simulink library "predictor_lib"  (R2016b)
settings: Solver=ode45  StartTime=0.0  StopTime=10.0  RelTol=1e-3  EnableMultiTasking=on
undefined symbols (not defined in the file): A_B_ISS_ISS, accel_bias, ase_of_num_aug, ase_total_num_states, ase_ts, gyro_bias, omega_B_ISS_B, P_EST_ISS_ISS, quat_ISS2B, tun_ase_max_accel, tun_ase_max_gyro, tun_ase_Q_imu, tun_ase_q_saturated_accel, tun_ase_q_saturated_gyro, V_B_ISS_ISS
libraries: math_utils x3
settings Model: Creator=jfusco1  LastModifiedBy=jfusco1
settings DataIOCC: LimitDataPoints=on  SaveFormat=Array
settings OptimizationCC: LifeSpan=inf
settings DebuggingCC: AllowSymbolicDim=off  SFUnexpectedBacktrackingDiag=warning  SFNoUnconditionalDefaultTransitionDiag=warning  SFExecutionAtInitializationDiag=none
settings HardwareCC: ProdBitPerPointer=32  ProdBitPerSizeT=32  ProdBitPerPtrDiffT=32  ProdLargestAtomicFloat=None  ProdIntDivRoundTo=Undefined  ProdEndianess=Unspecified  ProdWordSize=32  ProdHWDeviceType=32-bit Generic
settings ModelReferenceCC: PropagateSignalLabelsOutOfModel=off
settings GRTTargetCC: TargetLangStandard=C89/C90 (ANSI)  GeneratePreprocessorConditionals=Disable all
settings ConfigComp: CovMetricSettings=dw  CovHtmlReporting=on  CovSaveCumulativeToWorkspaceVar=on  CovSaveSingleToWorkspaceVar=on  CovExternalEMLEnable=off

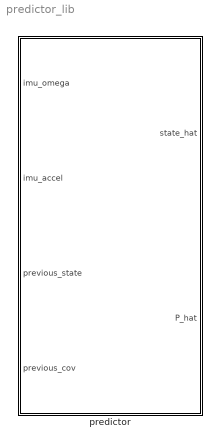
== system predictor_lib ==
  predictor : Subsystem

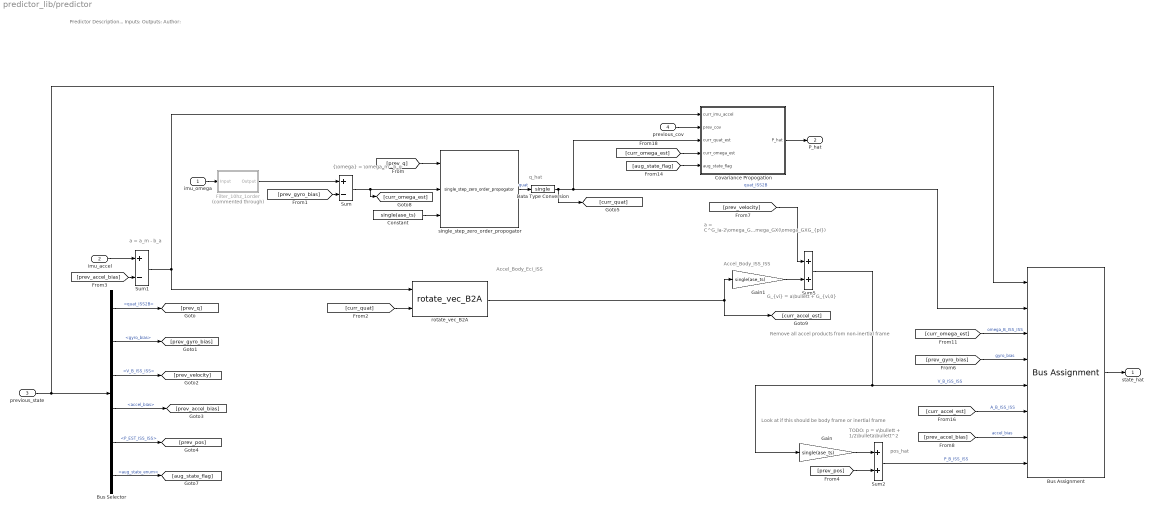
== system predictor_lib/predictor ==
  note: {\omega} = \omega_m - b_g
  note: Predictor
      | Description...
      |
      | Inputs:
      |
      | Outputs:
      |
      | Author:
  note: a = a_m - b_a
  note: q_hat
  note: TODO: p = v\bullett + 1/2\bulleta\bullett^2
  note: pos_hat
  note: a = C^G_Ia-2\omega_GXG_{vi}-\omega_GX(\omega_GXG_{pi})
  note: Accel_Body_Eci_ISS
  note: G_{vi} = a\bullett + G_{vi,0}
  note: Look at if this should be body frame or inertial frame
  note: Remove all accel products
      | from non-inertial frame
  note: Accel_Body_ISS_ISS
  imu_omega : Inport
  imu_accel : Inport  Port=2
  previous_state : Inport  Port=3
  previous_cov : Inport  Port=4
  Bus Assignment : BusAssignment  AssignedSignals=quat_ISS2B,omega_B_ISS_B,gyro_bias,V_B_ISS_ISS,A_B_ISS_ISS,accel_bias,P_EST_ISS_ISS
  Bus Selector : BusSelector  OutputSignals=quat_ISS2B,gyro_bias,V_B_ISS_ISS,accel_bias,P_EST_ISS_ISS,aug_state_enum
  Constant : Constant  Value=single(ase_ts)
  Covariance Propogation : Subsystem
  Data Type Conversion : DataTypeConversion  OutDataTypeStr=single
  Filter_10hz_1order : Subsystem  Tag=FilterWizardSubSystem  Commented=through
      settings: ErrorFcn=dspFilterRealizedInBasicElemsAlgLoopErrFcnCallback
  Gain : Gain  Gain=single(ase_ts)  OutDataTypeStr=single
  Gain1 : Gain  Gain=single(ase_ts)  OutDataTypeStr=single
  Sum : Sum  Inputs=+-
  Sum1 : Sum  Inputs=+-
  Sum2 : Sum
  Sum5 : Sum
  rotate_vec_B2A : math_utils/rotate_vec_B2A  SystemSampleTime=-1
  single_step_zero_order_propogator : math_utils/single_step_zero_order_propogator  SystemSampleTime=-1
  state_hat : Outport
  P_hat : Outport  Port=2
  wires:
  Bus Selector/4 -> [prev_accel_bias]  "<accel_bias>"
  Bus Selector/6 -> [aug_state_flag]  "<aug_state_enum>"
  Bus Assignment/1 -> state_hat/1
  imu_accel/1 -> Sum1/1
  Filter_10hz_1order/1(Output) -> Sum/1
  imu_omega/1 -> Filter_10hz_1order/1(Input)
  Sum/1 -> single_step_zero_order_propogator/2, [curr_omega_est]
  Constant/1 -> single_step_zero_order_propogator/3
  Gain/1 -> Sum2/1
  Sum1/1 -> rotate_vec_B2A/1, Covariance Propogation/1(curr_imu_accel)
  rotate_vec_B2A/1 -> Gain1/1, [curr_accel_est]
  Gain1/1 -> Sum5/2
  Bus Selector/1 -> [prev_q]  "<quat_ISS2B>"
  Bus Selector/2 -> [prev_gyro_bias]  "<gyro_bias>"
  Bus Selector/3 -> [prev_velocity]  "<V_B_ISS_ISS>"
  Bus Selector/5 -> [prev_pos]  "<P_EST_ISS_ISS>"
  [prev_q] -> single_step_zero_order_propogator/1
  [curr_quat] -> rotate_vec_B2A/2
  [prev_gyro_bias] -> Sum/2
  [prev_velocity] -> Sum5/1
  [prev_accel_bias] -> Sum1/2
  [prev_pos] -> Sum2/2
  single_step_zero_order_propogator/1 -> Data Type Conversion/1  "quat"
  [prev_accel_bias] -> Bus Assignment/7  "accel_bias"
  Sum2/1 -> Bus Assignment/8  "P_B_ISS_ISS"
  [prev_gyro_bias] -> Bus Assignment/4  "gyro_bias"
  Sum5/1 -> Bus Assignment/5, Gain/1  "V_B_ISS_ISS"
  Data Type Conversion/1 -> Covariance Propogation/3(curr_quat_est), Bus Assignment/2, [curr_quat]  "quat_ISS2B"
  previous_state/1 -> Bus Assignment/1, Bus Selector/1
  [curr_omega_est] -> Bus Assignment/3  "omega_B_ISS_ISS"
  [curr_accel_est] -> Bus Assignment/6  "A_B_ISS_ISS"
  previous_cov/1 -> Covariance Propogation/2(prev_cov)
  Covariance Propogation/1(P_hat) -> P_hat/1
  [curr_omega_est] -> Covariance Propogation/4(curr_omega_est)
  [aug_state_flag] -> Covariance Propogation/5(aug_state_flag)

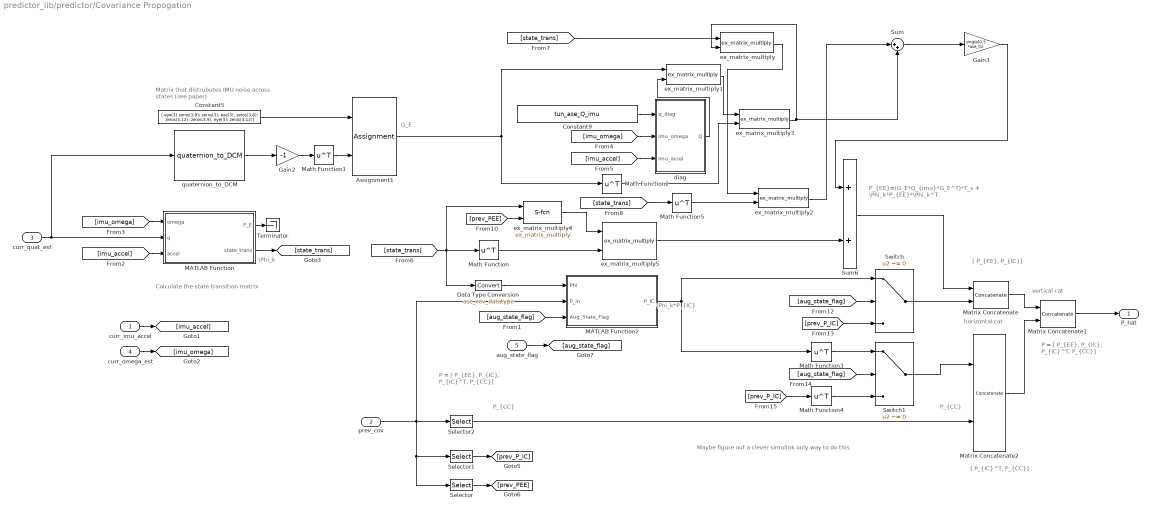
== system predictor_lib/predictor/Covariance Propogation ==
  note: P = [ P_{EE}, P_{IC};
      |
      |         P_{IC}^T, P_{CC}]
  note: \Phi_k
  note: G_E
  note: Matrix that distrubutes IMU noise across states (see paper)
  note: Calculate the state transition matrix
  note: P_{EE}=(G_E*Q_{imu}*G_E^T)*T_s + \Phi_k*P_{EE}*\Phi_k^T
  note: \Phi_k*P_{IC}
  note: P_{CC}
  note: P_{CC}
  note: [ P_{EE}, P_{IC}]
  note: [ P_{IC}^T, P_{CC}]
  note: P = [ P_{EE}, P_{IC};
      |
      |         P_{IC}^T, P_{CC}]
  note: horizontal cat
  note: vertical cat
  note: Maybe figure out a clever simulink only way to do this
  curr_imu_accel : Inport
  prev_cov : Inport  Port=2  OutDataTypeStr=ase_cov_datatype
  curr_quat_est : Inport  Port=3
  curr_omega_est : Inport  Port=4
  aug_state_flag : Inport  Port=5
  Assignment1 : Assignment  NumberOfDimensions=2  DiagnosticForDimensions=Warning  IndexOptions=Index vector (dialog),Index vector (dialog)  Indices=[7 8 9],[7 8 9]  OutputSizes=1,1
  Constant5 : Constant  Value=[-eye(3) zeros(3,9); zeros(3), eye(3), zeros(3,6); zeros(3,12); zeros(3,9), eye(3); zeros(3,12)]  OutDataTypeStr=ase_cov_datatype
  Constant9 : Constant  Value=tun_ase_Q_imu  OutDataTypeStr=ase_cov_datatype
  Data Type Conversion : DataTypeConversion  OutDataTypeStr=ase_cov_datatype
  Gain2 : Gain  Gain=-1  OutDataTypeStr=Inherit: Inherit via back propagation
  Gain3 : Gain  Gain=single(0.5 *ase_ts)
  MATLAB Function : MATLAB Function  TreatAsAtomicUnit=on
  MATLAB Function2 : MATLAB Function  TreatAsAtomicUnit=on
  Math Function{,1..5} (6 alike) : Math  Operator=transpose  SaturateOnIntegerOverflow=on
  Matrix Concatenate : Concatenate  Mode=Multidimensional array  ConcatenateDimension=2
  Matrix Concatenate1 : Concatenate  Mode=Multidimensional array
  Matrix Concatenate2 : Concatenate  Mode=Multidimensional array  ConcatenateDimension=2
  Selector : Selector  NumberOfDimensions=2  InputPortWidth=21  IndexOptions=Index vector (dialog),Index vector (dialog)  Indices=[1:15],[1:15]  OutputSizes=1,1
  Selector1 : Selector  NumberOfDimensions=2  InputPortWidth=21  IndexOptions=Index vector (dialog),Index vector (dialog)  Indices=[1:15],[16:ase_total_num_states]  OutputSizes=1,1
  Selector2 : Selector  NumberOfDimensions=2  InputPortWidth=21  IndexOptions=Index vector (dialog),Index vector (dialog)  Indices=[16:ase_total_num_states],[16:ase_total_num_states]  OutputSizes=1,1
  Sum : Sum  Inputs=|++
  Sum6 : Sum
  Switch : Switch  Criteria=u2 ~= 0
  Switch1 : Switch  Criteria=u2 ~= 0
  Terminator : Terminator
  diag : MATLAB Function  TreatAsAtomicUnit=on
  ex_matrix_multiply : S-Function  FunctionName=ex_matrix_multiply  SFunctionDeploymentMode=off  EnableBusSupport=off  mask(Legacy Function){SFunctionSpec=void matrix_multiply(single u1[][], int32 size(u1, 1), int32 size(u1, 2), single u2[][], int32 size(u2, 1), int32 size(u2, 2), single y1[size(u1, 1)][size(u2, 2)]), ShowSpec=off}
      mask prompts: ShowSpec "Display function specification"
      mask help:
      | This block allows you to call the legacy functions specified by the following Legacy Code Tool definition:
      | def.SFunctionName = 'ex_matrix_multiply';
      | def.OutputFcnSpec = 'void matrix_multiply(single u1[][], int32 size(u1, 1), int32 size(u1, 2), single u2[][], int32 size(u2, 1), int32 size(u2, 2), single y1[size(u1, 1)][size(u2, 2)])';
      | def.HeaderFiles = {'matrix_multiply.h'};
      | def.SourceFiles = {'matrix_multiply.cpp'};
      | def.IncPaths = {'cxx_functions/include', '/usr/include/eigen3'};
      | def.SrcPaths = {'cxx_functions/src', '/usr/include/eigen3/Eigen/src'};
      | def.Options.language = 'C++';
      mask Help: <p>This block was generated automatically by the Legacy Code Tool. For detailed help on this tool, call<a href="matlab:legacy_code('help')"> legacy_code('help')</a>.</p>
      mask Callback ShowSpec:
      | if strcmp(get_param(gcbh, 'ShowSpec'), 'on')
      |   set_param(gcbh, 'MaskDisplay', sprintf('fprintf(''%s'');', get_param(gcbh, 'SFunctionSpec')));
      | else
      |   set_param(gcbh, 'MaskDisplay', sprintf('fprintf(''%s'');', get_param(gcbh, 'FunctionName')));
      | end
      mask Display: fprintf('ex_matrix_multiply');
  ex_matrix_multiply1 : S-Function  FunctionName=ex_matrix_multiply  SFunctionDeploymentMode=off  EnableBusSupport=off  mask(Legacy Function){SFunctionSpec=void matrix_multiply(single u1[][], int32 size(u1, 1), int32 size(u1, 2), single u2[][], int32 size(u2, 1), int32 size(u2, 2), single y1[size(u1, 1)][size(u2, 2)]), ShowSpec=off}
      mask prompts: ShowSpec "Display function specification"
      mask help:
      | This block allows you to call the legacy functions specified by the following Legacy Code Tool definition:
      | def.SFunctionName = 'ex_matrix_multiply';
      | def.OutputFcnSpec = 'void matrix_multiply(single u1[][], int32 size(u1, 1), int32 size(u1, 2), single u2[][], int32 size(u2, 1), int32 size(u2, 2), single y1[size(u1, 1)][size(u2, 2)])';
      | def.HeaderFiles = {'matrix_multiply.h'};
      | def.SourceFiles = {'matrix_multiply.cpp'};
      | def.IncPaths = {'cxx_functions/include', '/usr/include/eigen3'};
      | def.SrcPaths = {'cxx_functions/src', '/usr/include/eigen3/Eigen/src'};
      | def.Options.language = 'C++';
      mask Help: <p>This block was generated automatically by the Legacy Code Tool. For detailed help on this tool, call<a href="matlab:legacy_code('help')"> legacy_code('help')</a>.</p>
      mask Callback ShowSpec:
      | if strcmp(get_param(gcbh, 'ShowSpec'), 'on')
      |   set_param(gcbh, 'MaskDisplay', sprintf('fprintf(''%s'');', get_param(gcbh, 'SFunctionSpec')));
      | else
      |   set_param(gcbh, 'MaskDisplay', sprintf('fprintf(''%s'');', get_param(gcbh, 'FunctionName')));
      | end
      mask Display: fprintf('ex_matrix_multiply');
  ex_matrix_multiply2 : S-Function  FunctionName=ex_matrix_multiply  SFunctionDeploymentMode=off  EnableBusSupport=off  mask(Legacy Function){SFunctionSpec=void matrix_multiply(single u1[][], int32 size(u1, 1), int32 size(u1, 2), single u2[][], int32 size(u2, 1), int32 size(u2, 2), single y1[size(u1, 1)][size(u2, 2)]), ShowSpec=off}
      mask prompts: ShowSpec "Display function specification"
      mask help:
      | This block allows you to call the legacy functions specified by the following Legacy Code Tool definition:
      | def.SFunctionName = 'ex_matrix_multiply';
      | def.OutputFcnSpec = 'void matrix_multiply(single u1[][], int32 size(u1, 1), int32 size(u1, 2), single u2[][], int32 size(u2, 1), int32 size(u2, 2), single y1[size(u1, 1)][size(u2, 2)])';
      | def.HeaderFiles = {'matrix_multiply.h'};
      | def.SourceFiles = {'matrix_multiply.cpp'};
      | def.IncPaths = {'cxx_functions/include', '/usr/include/eigen3'};
      | def.SrcPaths = {'cxx_functions/src', '/usr/include/eigen3/Eigen/src'};
      | def.Options.language = 'C++';
      mask Help: <p>This block was generated automatically by the Legacy Code Tool. For detailed help on this tool, call<a href="matlab:legacy_code('help')"> legacy_code('help')</a>.</p>
      mask Callback ShowSpec:
      | if strcmp(get_param(gcbh, 'ShowSpec'), 'on')
      |   set_param(gcbh, 'MaskDisplay', sprintf('fprintf(''%s'');', get_param(gcbh, 'SFunctionSpec')));
      | else
      |   set_param(gcbh, 'MaskDisplay', sprintf('fprintf(''%s'');', get_param(gcbh, 'FunctionName')));
      | end
      mask Display: fprintf('ex_matrix_multiply');
  ex_matrix_multiply3 : S-Function  FunctionName=ex_matrix_multiply  SFunctionDeploymentMode=off  EnableBusSupport=off  mask(Legacy Function){SFunctionSpec=void matrix_multiply(single u1[][], int32 size(u1, 1), int32 size(u1, 2), single u2[][], int32 size(u2, 1), int32 size(u2, 2), single y1[size(u1, 1)][size(u2, 2)]), ShowSpec=off}
      mask prompts: ShowSpec "Display function specification"
      mask help:
      | This block allows you to call the legacy functions specified by the following Legacy Code Tool definition:
      | def.SFunctionName = 'ex_matrix_multiply';
      | def.OutputFcnSpec = 'void matrix_multiply(single u1[][], int32 size(u1, 1), int32 size(u1, 2), single u2[][], int32 size(u2, 1), int32 size(u2, 2), single y1[size(u1, 1)][size(u2, 2)])';
      | def.HeaderFiles = {'matrix_multiply.h'};
      | def.SourceFiles = {'matrix_multiply.cpp'};
      | def.IncPaths = {'cxx_functions/include', '/usr/include/eigen3'};
      | def.SrcPaths = {'cxx_functions/src', '/usr/include/eigen3/Eigen/src'};
      | def.Options.language = 'C++';
      mask Help: <p>This block was generated automatically by the Legacy Code Tool. For detailed help on this tool, call<a href="matlab:legacy_code('help')"> legacy_code('help')</a>.</p>
      mask Callback ShowSpec:
      | if strcmp(get_param(gcbh, 'ShowSpec'), 'on')
      |   set_param(gcbh, 'MaskDisplay', sprintf('fprintf(''%s'');', get_param(gcbh, 'SFunctionSpec')));
      | else
      |   set_param(gcbh, 'MaskDisplay', sprintf('fprintf(''%s'');', get_param(gcbh, 'FunctionName')));
      | end
      mask Display: fprintf('ex_matrix_multiply');
  ex_matrix_multiply4 : S-Function  FunctionName=ex_matrix_multiply  SFunctionDeploymentMode=off  EnableBusSupport=off  mask(Legacy Function){SFunctionSpec=void matrix_multiply(single u1[][], int32 size(u1, 1), int32 size(u1, 2), single u2[][], int32 size(u2, 1), int32 size(u2, 2), single y1[size(u1, 1)][size(u2, 2)]), ShowSpec=off}
      mask prompts: ShowSpec "Display function specification"
      mask help:
      | This block allows you to call the legacy functions specified by the following Legacy Code Tool definition:
      | def.SFunctionName = 'ex_matrix_multiply';
      | def.OutputFcnSpec = 'void matrix_multiply(single u1[][], int32 size(u1, 1), int32 size(u1, 2), single u2[][], int32 size(u2, 1), int32 size(u2, 2), single y1[size(u1, 1)][size(u2, 2)])';
      | def.HeaderFiles = {'matrix_multiply.h'};
      | def.SourceFiles = {'matrix_multiply.cpp'};
      | def.IncPaths = {'cxx_functions/include', '/usr/include/eigen3'};
      | def.SrcPaths = {'cxx_functions/src', '/usr/include/eigen3/Eigen/src'};
      | def.Options.language = 'C++';
      mask Help: <p>This block was generated automatically by the Legacy Code Tool. For detailed help on this tool, call<a href="matlab:legacy_code('help')"> legacy_code('help')</a>.</p>
      mask Callback ShowSpec:
      | if strcmp(get_param(gcbh, 'ShowSpec'), 'on')
      |   set_param(gcbh, 'MaskDisplay', sprintf('fprintf(''%s'');', get_param(gcbh, 'SFunctionSpec')));
      | else
      |   set_param(gcbh, 'MaskDisplay', sprintf('fprintf(''%s'');', get_param(gcbh, 'FunctionName')));
      | end
      mask Display: fprintf('ex_matrix_multiply');
  ex_matrix_multiply5 : S-Function  FunctionName=ex_matrix_multiply  SFunctionDeploymentMode=off  EnableBusSupport=off  mask(Legacy Function){SFunctionSpec=void matrix_multiply(single u1[][], int32 size(u1, 1), int32 size(u1, 2), single u2[][], int32 size(u2, 1), int32 size(u2, 2), single y1[size(u1, 1)][size(u2, 2)]), ShowSpec=off}
      mask prompts: ShowSpec "Display function specification"
      mask help:
      | This block allows you to call the legacy functions specified by the following Legacy Code Tool definition:
      | def.SFunctionName = 'ex_matrix_multiply';
      | def.OutputFcnSpec = 'void matrix_multiply(single u1[][], int32 size(u1, 1), int32 size(u1, 2), single u2[][], int32 size(u2, 1), int32 size(u2, 2), single y1[size(u1, 1)][size(u2, 2)])';
      | def.HeaderFiles = {'matrix_multiply.h'};
      | def.SourceFiles = {'matrix_multiply.cpp'};
      | def.IncPaths = {'cxx_functions/include', '/usr/include/eigen3'};
      | def.SrcPaths = {'cxx_functions/src', '/usr/include/eigen3/Eigen/src'};
      | def.Options.language = 'C++';
      mask Help: <p>This block was generated automatically by the Legacy Code Tool. For detailed help on this tool, call<a href="matlab:legacy_code('help')"> legacy_code('help')</a>.</p>
      mask Callback ShowSpec:
      | if strcmp(get_param(gcbh, 'ShowSpec'), 'on')
      |   set_param(gcbh, 'MaskDisplay', sprintf('fprintf(''%s'');', get_param(gcbh, 'SFunctionSpec')));
      | else
      |   set_param(gcbh, 'MaskDisplay', sprintf('fprintf(''%s'');', get_param(gcbh, 'FunctionName')));
      | end
      mask Display: fprintf('ex_matrix_multiply');
  quaternion_to_DCM : math_utils/quaternion_to_DCM  SystemSampleTime=-1
  P_hat : Outport  OutDataTypeStr=ase_cov_datatype
  wires:
  ex_matrix_multiply1/1 -> ex_matrix_multiply3/1
  ex_matrix_multiply4/1 -> ex_matrix_multiply5/1
  Math Function5/1 -> ex_matrix_multiply2/2
  [state_trans] -> Math Function5/1
  [state_trans] -> ex_matrix_multiply/1
  [state_trans] -> Math Function/1, Data Type Conversion/1, ex_matrix_multiply4/1
  MATLAB Function/2(state_trans) -> [state_trans]
  [imu_accel] -> diag/3(imu_accel)
  [imu_omega] -> diag/2(imu_omega)
  [imu_omega] -> MATLAB Function/1(omega)
  curr_omega_est/1 -> [imu_omega]
  [imu_accel] -> MATLAB Function/3(accel)
  curr_imu_accel/1 -> [imu_accel]
  diag/1(Q) -> ex_matrix_multiply1/2
  Data Type Conversion/1 -> MATLAB Function2/1(Phi)
  prev_cov/1 -> Selector/1, Selector1/1, Selector2/1, MATLAB Function2/2(P_in)
  [aug_state_flag] -> MATLAB Function2/3(Aug_State_Flag)
  [prev_P_IC] -> Switch/3
  Matrix Concatenate2/1 -> Matrix Concatenate1/2
  Selector/1 -> [prev_PEE]
  [aug_state_flag] -> Switch1/2
  Selector2/1 -> Matrix Concatenate2/2
  Selector1/1 -> [prev_P_IC]
  [aug_state_flag] -> Switch/2
  MATLAB Function2/1(P_IC) -> Switch/1, Math Function3/1
  ex_matrix_multiply3/1 -> Sum/2, ex_matrix_multiply/2
  Matrix Concatenate/1 -> Matrix Concatenate1/1
  Matrix Concatenate1/1 -> P_hat/1
  Switch/1 -> Matrix Concatenate/2
  Switch1/1 -> Matrix Concatenate2/1
  Math Function3/1 -> Switch1/1
  Constant5/1 -> Assignment1/1
  Sum6/1 -> Matrix Concatenate/1
  Assignment1/1 -> Math Function2/1, ex_matrix_multiply1/1
  Constant9/1 -> diag/1(q_diag)
  ex_matrix_multiply5/1 -> Sum6/2
  Gain2/1 -> Math Function1/1
  Math Function1/1 -> Assignment1/2
  quaternion_to_DCM/1 -> Gain2/1
  Math Function/1 -> ex_matrix_multiply5/2
  [prev_PEE] -> ex_matrix_multiply4/2
  MATLAB Function/1(F_E) -> Terminator/1
  curr_quat_est/1 -> quaternion_to_DCM/1, MATLAB Function/2(q)
  [prev_P_IC] -> Math Function4/1
  Math Function4/1 -> Switch1/3
  aug_state_flag/1 -> [aug_state_flag]
  Math Function2/1 -> ex_matrix_multiply3/2
  ex_matrix_multiply/1 -> ex_matrix_multiply2/1
  ex_matrix_multiply2/1 -> Sum/1
  Sum/1 -> Gain3/1
  Gain3/1 -> Sum6/1

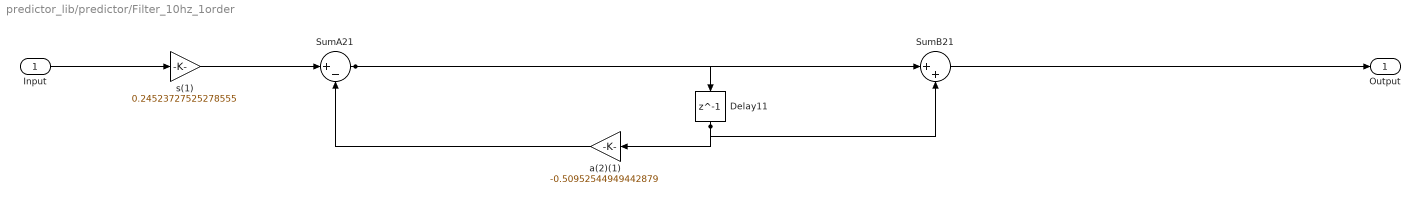
== system predictor_lib/predictor/Filter_10hz_1order ==
  Input : Inport
  Delay11 : Delay  DelayLength=1  InitialCondition=0
  SumA21 : Sum  Inputs=|+-  RndMeth=Nearest  SaturateOnIntegerOverflow=on  OutDataTypeStr=Inherit: Same as first input
  SumB21 : Sum  Inputs=|++  RndMeth=Nearest  SaturateOnIntegerOverflow=on  OutDataTypeStr=Inherit: Same as first input
  a(2)(1) : Gain  Gain=-0.50952544949442879  ParamDataTypeStr=double  RndMeth=Nearest  SaturateOnIntegerOverflow=on  OutDataTypeStr=Inherit: Same as input
  s(1) : Gain  Gain=0.24523727525278555  ParamDataTypeStr=double  RndMeth=Nearest  SaturateOnIntegerOverflow=on  OutDataTypeStr=Inherit: Same as input
  Output : Outport
  wires:
  Delay11/1 -> SumB21/2, a(2)(1)/1
  a(2)(1)/1 -> SumA21/2
  SumB21/1 -> Output/1
  SumA21/1 -> Delay11/1, SumB21/1
  s(1)/1 -> SumA21/1
  Input/1 -> s(1)/1

== matlab function predictor_lib/predictor/Covariance Propogation/diag ==
  data: q_diag input size=12; Q output size=[12 12]; imu_omega input; imu_accel input; tun_ase_max_gyro parameter; tun_ase_max_accel parameter; tun_ase_q_saturated_gyro parameter; tun_ase_q_saturated_accel parameter
function Q = create_q_imu(q_diag, imu_omega, imu_accel, tun_ase_max_gyro, tun_ase_max_accel, tun_ase_q_saturated_gyro, tun_ase_q_saturated_accel)
%#codegen
q_diag(abs([imu_omega' 0 0 0 0 0 0 0 0 0]) >= tun_ase_max_gyro)  = tun_ase_q_saturated_gyro;
q_diag(abs([0 0 0 0 0 0 imu_accel' 0 0 0]) >= tun_ase_max_accel) = tun_ase_q_saturated_accel;
Q = diag(q_diag);

end

== matlab function predictor_lib/predictor/Covariance Propogation/MATLAB Function ==
  data: omega input; q input; accel input; F_E output; state_trans output; ase_ts parameter
function [F_E, state_trans]  = fcn(omega, q, accel, ase_ts)
%#codegen

  S = [0 -q(3)  q(2);
       q(3)     0 -q(1);
      -q(2)  q(1)     0]; 
  a = [q(4) * eye(3, 3) - S; -q(1:3)'];
  b = [q(4) * eye(3, 3) + S; -q(1:3)'];
  C = b' * a;

  skew_mat_omega = [0 -omega(3)  omega(2);
       omega(3)     0 -omega(1);
      -omega(2)  omega(1)     0];
  
  accel = abs(accel);
    skew_mat_accel = [0 -accel(3)  accel(2);
       accel(3)     0 -accel(1);
      -accel(2)  accel(1)     0];
  
  I = eye(3, 'single');
  z = zeros(3, 'single');
  
  F_E = [-skew_mat_omega -I z                  z     z;
                    z  z z                  z     z;
        -C' * skew_mat_accel  z z (-C') z;
                    z  z z                  z     z;
                    z  z I                  z     z];
  
%state_trans_1 = single(eye(15) + F_E*0.01); % Consider using expm


state_trans = single(expm(F_E*ase_ts)); % Paramaterize Ts

== matlab function predictor_lib/predictor/Covariance Propogation/MATLAB Function2 ==
  data: Phi input; P_in input; P_IC output ase_cov_datatype; Aug_State_Flag input; ase_total_num_states parameter; ase_of_num_aug parameter
function P_IC   = fcn(Phi, P_in, Aug_State_Flag, ase_total_num_states, ase_of_num_aug)
%#codegen

  P_IC = P_in(1:15, 16:ase_total_num_states); % Extract the cross coupled part of the camera and IMU covariance
  
  % Creates a matrix where each column is the indices for each augmentation
  Aug_Indx = reshape(1:(ase_of_num_aug+1)*6, 6,(ase_of_num_aug+1)); % Number of columns is number of OF augmentations + ML augmentations
  % Collect the indices of the valid current augmentations
  
  % Form a vector with the valid indices corresponding to the current
  % number of augmentations
 valid_indx_mat = Aug_Indx(:,logical(bitget(Aug_State_Flag, 1:ase_of_num_aug+1)));
 valid_col = valid_indx_mat(:);
 
 % Do the covariance propagation
 P_IC(1:15, valid_col) = Phi * P_in(1:15, 15+valid_col);
  
  %Aug_Indx(Aug_State_Flag)
 
  % Do the multiplication with current valid indices
  
  %P(:, D+1:size(P, 2)) = Phi * P(1:D, D+1:size(P, 2));
